simulink model "for_report"  (R2023b)
settings: Solver=ode8  StartTime=0.0  StopTime=30  FixedStep=t_step  MaxStep=1e-6  RelTol=1e-6
values from neighbouring files (symbols this model uses):
  A = 0.012456    [Compute_TFs_and_StateSpace.m]    (also in parameters.m)
  C_l = k_c    (= 8.37005e-08)    [parameters.m]
  k_c = k_pl/2    (= 8.37005e-08)    [parameters.m]
  K_h = 4*beta_e*A^2/V_t    (= 45213.1716837)    [parameters.m]
  k_q = 1934.50    (= 1934.5)    [parameters.m]
  k_sv = 1934.50    (= 1934.5)    [parameters.m]
  tau_sv = 0.0246    [Compute_TFs_and_StateSpace.m]    (also in parameters.m)
libraries: cstblocks x1
settings Model: Creator=afons  LastModifiedBy=afons

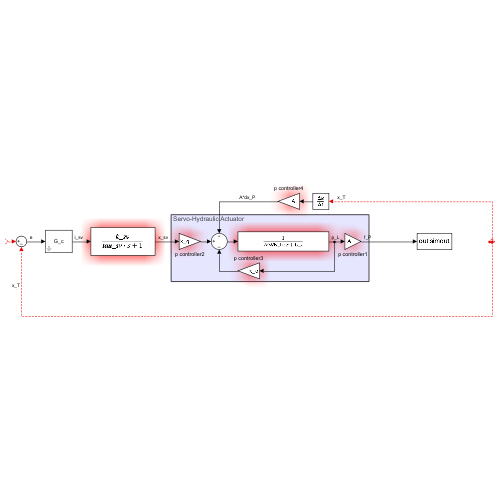
[thumbnail: Simulink's stored preview of the top-level diagram]
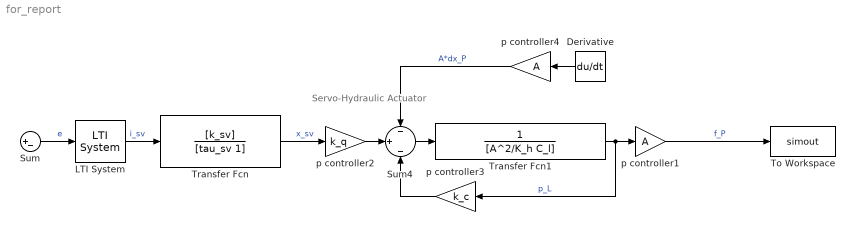
== system for_report ==
  note: Servo-Hydraulic Actuator
  Derivative : Derivative
  LTI System : cstblocks/LTI System  sys=tf(1,[1 1])  IC=[]  PadeOrder=0
  Sum : Sum  Inputs=|+-
  Sum4 : Sum  Inputs=-|+|-
  To Workspace : ToWorkspace  VariableName=simout  SaveFormat=Timeseries  SampleTime=-1
  Transfer Fcn : TransferFcn  Numerator=[k_sv]  Denominator=[tau_sv 1]
  Transfer Fcn1 : TransferFcn  Denominator=[A^2/K_h C_l]
  p controller1 : Gain  Gain=A
  p controller2 : Gain  Gain=k_q
  p controller3 : Gain  Gain=k_c
  p controller4 : Gain  Gain=A
  wires:
  Sum/1 -> LTI System/1  "e"
  LTI System/1 -> Transfer Fcn/1  "i_sv"
  Transfer Fcn/1 -> p controller2/1  "x_sv"
  Sum4/1 -> Transfer Fcn1/1
  p controller4/1 -> Sum4/1  "A*dx_P"
  Transfer Fcn1/1 -> p controller1/1, p controller3/1  "p_L"
  p controller1/1 -> To Workspace/1  "f_P"
  ? -> Sum/2, Derivative/1  "x_T"
  p controller2/1 -> Sum4/2
  p controller3/1 -> Sum4/3
  Derivative/1 -> p controller4/1
  ? -> Sum/1
